simulink model "simSystem_v1"  (R2021b)
settings: Solver=VariableStepAuto  StartTime=0.0  StopTime=30  RelTol=1e-3
InitFcn:
  | initFcn
StopFcn:
  | stopFcn
values from neighbouring files (symbols this model uses):
  D_LIN = 1    [initFcn.m]
  D_QUAD = 1    [initFcn.m]
  M = M_RB + M_A    [initFcn.m]
  range = 2    [initFcn.m]
undefined symbols (not defined in the file or in its folder): B, I0, m, M_A, p, r_b_b, r_g_b, T
libraries: simulink x2, cstblocks x2, slpidlib x2, aerolibguid x1
settings Model: Creator=User  LastModifiedBy=saigon

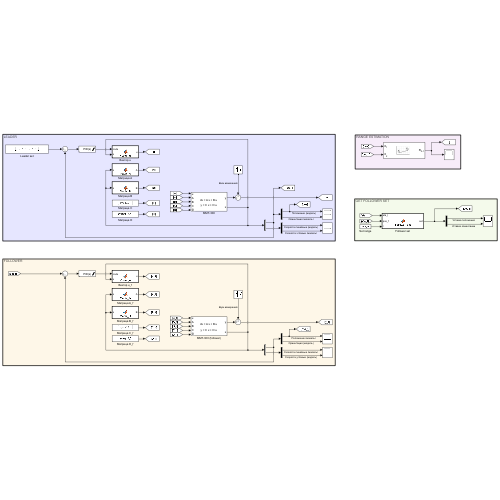
[thumbnail: Simulink's stored preview of the top-level diagram]
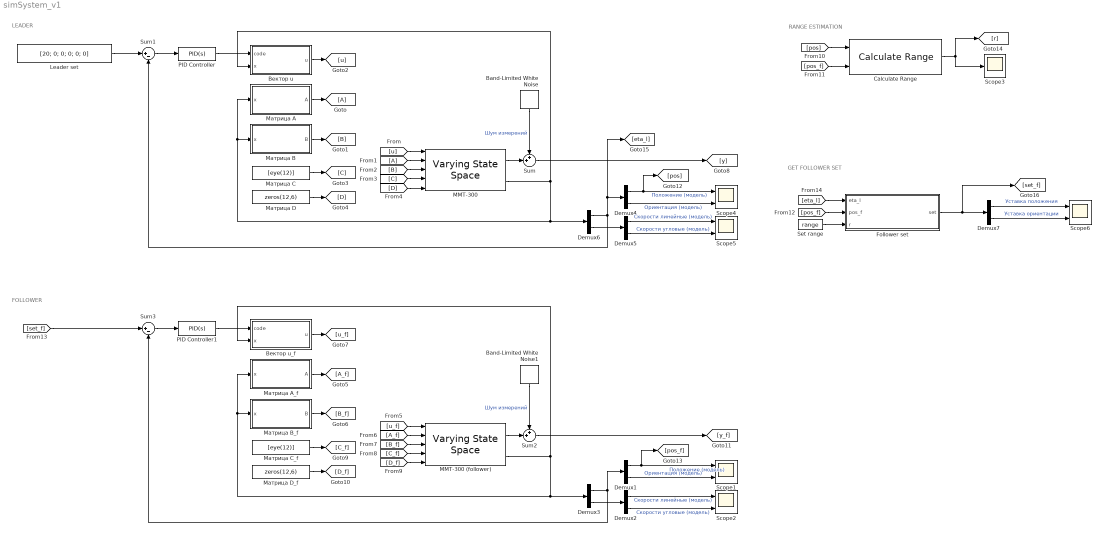
== system simSystem_v1 ==
  note: GET FOLLOWER SET
  note: RANGE ESTIMATION
  note: LEADER
  note: FOLLOWER
  Band-Limited White Noise : simulink/Sources/Band-Limited White Noise  Cov=[0.00000]  Ts=0.1  seed=[23341]
  Band-Limited White Noise1 : simulink/Sources/Band-Limited White Noise  Cov=[0.00000]  Ts=0.1  seed=[23341]
  Calculate Range : aerolibguid/Calculate Range
      settings: SourceProductBaseCode=AE
  Demux{1..7} (7 alike) : Demux  Outputs=2
  Follower set : MATLAB Function  TreatAsAtomicUnit=on
  Leader set : Constant  Value=[20; 0; 0; 0; 0; 0]
  MMT-300 : cstblocks/Linear Parameter Varying/Varying State Space  x0=zeros(12,1)  xNames=''  OutputX=on  OutputDX=off
  MMT-300 (follower) : cstblocks/Linear Parameter Varying/Varying State Space  x0=[-5;-5;0;0;0;0;zeros(6,1)]  xNames=''  OutputX=on  OutputDX=off
  PID Controller : slpidlib/PID Controller  Controller=PID  Form=Parallel  TimeDomain=Continuous-time  UseExternalTs=off  SampleTime=-1  IntegratorMethod=Forward Euler  FilterMethod=Forward Euler  ControllerParametersSource=internal  P=[100; 100; 100; 1500; 1500; 1500]  I=[0.5; 0.5; 0.5; 1; 1; 1]  D=[300; 300; 300; 400; 400; 400]  UseFilter=on  N=100  TunerSelectOption=Transfer Function Based (PID Tuner App)  InitialConditionSource=internal  InitialConditionForIntegrator=0  InitialConditionForFilter=0  DifferentiatorICPrevScaledInput=0  ExternalReset=none  TrackingMode=off  Kt=1  LimitOutput=on  SatLimitsSource=internal  UpperSaturationLimit=1000  LowerSaturationLimit=-1000  LinearizeAsGain=on  AntiWindupMode=none  Kb=1  POutMin=[]  POutMax=[]  IOutMin=[]  IOutMax=[]  DOutMin=[]  DOutMax=[]  NOutMin=[]  NOutMax=[]  SumOutMin=[]  SumOutMax=[]  SaturationOutMin=[]  SaturationOutMax=[]  PParamMin=[]  PParamMax=[]  IParamMin=[]  IParamMax=[]  DParamMin=[]  DParamMax=[]  NParamMin=[]  NParamMax=[]  KbParamMin=[]  KbParamMax=[]  KtParamMin=[]  KtParamMax=[]  KbOutMin=[]  KbOutMax=[]  KtOutMin=[]  KtOutMax=[]  IntegratorOutMin=[]  IntegratorOutMax=[]  FilterOutMin=[]  FilterOutMax=[]  SumI1OutMin=[]  SumI1OutMax=[]  SumI2OutMin=[]  SumI2OutMax=[]  SumI3OutMin=[]  SumI3OutMax=[]  SumI4OutMin=[]  SumI4OutMax=[]  SumDOutMin=[]  SumDOutMax=[]  DifferentiatorOutMin=[]  DifferentiatorOutMax=[]  FilterDiffOutCoefMin=[]  FilterDiffOutCoefMax=[]  ReciprocalOutMin=[]  ReciprocalOutMax=[]  SumDenOutMin=[]  SumDenOutMax=[]  SumNumOutMin=[]  SumNumOutMax=[]  DivideOutMin=[]  DivideOutMax=[]  UdiffTsProdOutMin=[]  UdiffTsProdOutMax=[]  NTsProdOutMin=[]  NTsProdOutMax=[]  UintegralTsProdOutMin=[]  UintegralTsProdOutMax=[]  UngainTsProdOutMin=[]  UngainTsProdOutMax=[]  IntegratorContinuousStateAttributes=''  IntegratorStateMustResolveToSignalObject=off  IntegratorRTWStateStorageClass=Auto  FilterContinuousStateAttributes=''  FilterStateMustResolveToSignalObject=off  FilterRTWStateStorageClass=Auto  ParallelPVariant=InternalParameters  IdealPVariant=Disabled  IVariant=InternalParameters  DVariant=InternalParameters  IntegratorVariant=Continuous  SatVariant=Enabled  AWVariant=Passthrough  PCopyVariant=Disabled  TRVariant=Disabled  FdbkBlocksVariant=Forward  IdealPFdbkVariant=Disabled  SatFdbkVariant=Disabled  DerivativeFilterVariant=ContFilter  NVariant=InternalParameters  NCopyVariant=Disabled  FilterICVariant=InternalICsFilter  IntegratorICVariant=InternalICs  ExternalResetVariant=Disabled  TRSumVariant=Passthrough  SumFdbkVariant=Disabled  SumVariant=Sum_PID  TsampFilterVariant=InternalTs  TsampNgainVariant=Passthrough  TsampIntegralVariant=Passthrough  ExternalSaturationOutDataTypeStr=Inherit: Same as second input
  PID Controller1 : slpidlib/PID Controller  Controller=PID  Form=Parallel  TimeDomain=Continuous-time  UseExternalTs=off  SampleTime=-1  IntegratorMethod=Forward Euler  FilterMethod=Forward Euler  ControllerParametersSource=internal  P=[100; 100; 100; 1500; 1500; 1500]  I=[0.5; 0.5; 0.5; 1; 1; 1]  D=[300; 300; 300; 400; 400; 400]  UseFilter=on  N=100  TunerSelectOption=Transfer Function Based (PID Tuner App)  InitialConditionSource=internal  InitialConditionForIntegrator=0  InitialConditionForFilter=0  DifferentiatorICPrevScaledInput=0  ExternalReset=none  TrackingMode=off  Kt=1  LimitOutput=on  SatLimitsSource=internal  UpperSaturationLimit=1000  LowerSaturationLimit=-1000  LinearizeAsGain=on  AntiWindupMode=none  Kb=1  POutMin=[]  POutMax=[]  IOutMin=[]  IOutMax=[]  DOutMin=[]  DOutMax=[]  NOutMin=[]  NOutMax=[]  SumOutMin=[]  SumOutMax=[]  SaturationOutMin=[]  SaturationOutMax=[]  PParamMin=[]  PParamMax=[]  IParamMin=[]  IParamMax=[]  DParamMin=[]  DParamMax=[]  NParamMin=[]  NParamMax=[]  KbParamMin=[]  KbParamMax=[]  KtParamMin=[]  KtParamMax=[]  KbOutMin=[]  KbOutMax=[]  KtOutMin=[]  KtOutMax=[]  IntegratorOutMin=[]  IntegratorOutMax=[]  FilterOutMin=[]  FilterOutMax=[]  SumI1OutMin=[]  SumI1OutMax=[]  SumI2OutMin=[]  SumI2OutMax=[]  SumI3OutMin=[]  SumI3OutMax=[]  SumI4OutMin=[]  SumI4OutMax=[]  SumDOutMin=[]  SumDOutMax=[]  DifferentiatorOutMin=[]  DifferentiatorOutMax=[]  FilterDiffOutCoefMin=[]  FilterDiffOutCoefMax=[]  ReciprocalOutMin=[]  ReciprocalOutMax=[]  SumDenOutMin=[]  SumDenOutMax=[]  SumNumOutMin=[]  SumNumOutMax=[]  DivideOutMin=[]  DivideOutMax=[]  UdiffTsProdOutMin=[]  UdiffTsProdOutMax=[]  NTsProdOutMin=[]  NTsProdOutMax=[]  UintegralTsProdOutMin=[]  UintegralTsProdOutMax=[]  UngainTsProdOutMin=[]  UngainTsProdOutMax=[]  IntegratorContinuousStateAttributes=''  IntegratorStateMustResolveToSignalObject=off  IntegratorRTWStateStorageClass=Auto  FilterContinuousStateAttributes=''  FilterStateMustResolveToSignalObject=off  FilterRTWStateStorageClass=Auto  ParallelPVariant=InternalParameters  IdealPVariant=Disabled  IVariant=InternalParameters  DVariant=InternalParameters  IntegratorVariant=Continuous  SatVariant=Enabled  AWVariant=Passthrough  PCopyVariant=Disabled  TRVariant=Disabled  FdbkBlocksVariant=Forward  IdealPFdbkVariant=Disabled  SatFdbkVariant=Disabled  DerivativeFilterVariant=ContFilter  NVariant=InternalParameters  NCopyVariant=Disabled  FilterICVariant=InternalICsFilter  IntegratorICVariant=InternalICs  ExternalResetVariant=Disabled  TRSumVariant=Passthrough  SumFdbkVariant=Disabled  SumVariant=Sum_PID  TsampFilterVariant=InternalTs  TsampNgainVariant=Passthrough  TsampIntegralVariant=Passthrough  ExternalSaturationOutDataTypeStr=Inherit: Same as second input
  Scope{1..2,4..6} (5 alike) : Scope  NumInputPorts=2
  Scope3 : Scope
  Set range : Constant  Value=range
  Sum : Sum  Inputs=++|
  Sum1 : Sum  Inputs=|+-
  Sum2 : Sum  Inputs=++|
  Sum3 : Sum  Inputs=|+-
  Вектор u : MATLAB Function  TreatAsAtomicUnit=on
  Вектор u_f : MATLAB Function  TreatAsAtomicUnit=on
  Матрица A : MATLAB Function  TreatAsAtomicUnit=on
  Матрица A_f : MATLAB Function  TreatAsAtomicUnit=on
  Матрица B : MATLAB Function  TreatAsAtomicUnit=on
  Матрица B_f : MATLAB Function  TreatAsAtomicUnit=on
  Матрица C : Constant  Value=[eye(12)]
  Матрица C_f : Constant  Value=[eye(12)]
  Матрица D : Constant  Value=zeros(12,6)
  Матрица D_f : Constant  Value=zeros(12,6)
  wires:
  MMT-300/1 -> Sum/2
  Band-Limited White Noise/1 -> Sum/1  "Шум измерений"
  Demux4/1 -> [pos], Scope4/1  "Положение (модель)"
  Demux4/2 -> Scope4/2  "Ориентация (модель)"
  Demux5/2 -> Scope5/2  "Скорости угловые (модель)"
  Demux5/1 -> Scope5/1  "Скорости линейные (модель)"
  Demux6/2 -> Demux5/1
  Матрица A/1(A) -> [A]
  Матрица B/1(B) -> [B]
  Вектор u/1(u) -> [u]
  Матрица C/1 -> [C]
  Матрица D/1 -> [D]
  [u] -> MMT-300/1
  [A] -> MMT-300/2
  [B] -> MMT-300/3
  [C] -> MMT-300/4
  [D] -> MMT-300/5
  MMT-300/2 -> Demux6/1, Матрица A/1(x), Матрица B/1(x), Вектор u/2(x)
  Sum/1 -> [y]
  Leader set/1 -> Sum1/1
  PID Controller/1 -> Вектор u/1(code)
  Sum1/1 -> PID Controller/1
  Sum3/1 -> PID Controller1/1
  PID Controller1/1 -> Вектор u_f/1(code)
  [set_f] -> Sum3/1
  Sum2/1 -> [y_f]
  MMT-300 (follower)/2 -> Вектор u_f/2(x), Матрица B_f/1(x), Матрица A_f/1(x), Demux3/1
  [D_f] -> MMT-300 (follower)/5
  [C_f] -> MMT-300 (follower)/4
  [B_f] -> MMT-300 (follower)/3
  [A_f] -> MMT-300 (follower)/2
  [u_f] -> MMT-300 (follower)/1
  Матрица D_f/1 -> [D_f]
  Матрица C_f/1 -> [C_f]
  Вектор u_f/1(u) -> [u_f]
  Матрица B_f/1(B) -> [B_f]
  Матрица A_f/1(A) -> [A_f]
  Demux3/1 -> Demux1/1, Sum3/2
  Demux3/2 -> Demux2/1
  Demux2/1 -> Scope2/1  "Скорости линейные (модель)"
  Demux2/2 -> Scope2/2  "Скорости угловые (модель)"
  Demux1/2 -> Scope1/2  "Ориентация (модель)"
  Demux1/1 -> [pos_f], Scope1/1  "Положение (модель)"
  Band-Limited White Noise1/1 -> Sum2/1  "Шум измерений"
  MMT-300 (follower)/1 -> Sum2/2
  [pos] -> Calculate Range/1
  [pos_f] -> Calculate Range/2
  Calculate Range/1 -> [r], Scope3/1
  [pos_f] -> Follower set/2(pos_f)
  Set range/1 -> Follower set/3(r)
  Demux6/1 -> Sum1/2, [eta_l], Demux4/1
  [eta_l] -> Follower set/1(eta_l)
  Follower set/1(set) -> [set_f], Demux7/1
  Demux7/2 -> Scope6/2  "Уставка ориентации"
  Demux7/1 -> Scope6/1  "Уставка положения"

== matlab function simSystem_v1/Вектор u_f ==
  data: code input [-127..127]; x input size=12; u output size=6; T parameter; p parameter; B parameter; m parameter; r_g_b parameter; r_b_b parameter
function u = Vector_u(code, x, T, p, B, m, r_g_b, r_b_b)
n = 6;
eta = x(1:n); 

%% РАСЧЕТ g(n)
x_g = r_g_b(1); y_g = r_g_b(2); z_g = r_g_b(3);
x_b = r_b_b(1); y_b = r_b_b(2); z_b = r_b_b(3);
g = @(eta)[ (m*9.81-B)*sin(eta(5)); 
           -(m*9.81-B)*cos(eta(5))*sin(eta(4)); 
           -(m*9.81-B)*cos(eta(5))*cos(eta(4));
           -(y_g*m*9.81-y_b*B)*cos(eta(5))*cos(eta(4)) + ...
              (z_g*m*9.81-z_b*B)*cos(eta(5))*sin(eta(4));
            (z_g*m*9.81-z_b*B)*sin(eta(5)) + ...
              (x_g*m*9.81-x_b*B)*cos(eta(5))*cos(eta(4));
           -(x_g*m*9.81-x_b*B)*cos(eta(5))*sin(eta(4)) - ...
              (y_g*m*9.81-y_b*B)*sin(eta(5)) ]; 


F = @(code)polyval(p,code);

f1 = @(code)[ F(code)*cos(deg2rad(22)); 
              0; 
              F(code)*sin(deg2rad(22)) ];
f2 = @(code)[ F(code)*cos(deg2rad(22)); 
              F(code)*sin(deg2rad(22));
              0 ];
f3 = @(code)[ F(code)*cos(deg2rad(22)); 
              0; 
              -F(code)*sin(deg2rad(22)) ];
f4 = @(code)[ F(code)*cos(deg2rad(22));  
              -F(code)*sin(deg2rad(22));
              0 ];
f5 = @(code)[ 0; 
              F(code); 
              0 ];
f6 = @(code)[ 0; 
              0; 
              -F(code) ];

r1 = T(1,:)'; 
r2 = T(2,:)'; 
r3 = T(3,:)';
r4 = T(4,:)';
r5 = T(5,:)';
r6 = T(6,:)';
tau1 = @(code)[ f1(code); cross(r1, f1(code)) ];
tau2 = @(code)[ f2(code); cross(r2, f2(code)) ];
tau3 = @(code)[ f3(code); cross(r3, f3(code)) ];
tau4 = @(code)[ f4(code); cross(r4, f4(code)) ];
tau5 = @(code)[ f5(code); cross(r5, f5(code)) ];
tau6 = @(code)[ f6(code); cross(r6, f6(code)) ];

tau_c = @(code)[ tau1(code(1)), tau2(code(2)), tau3(code(3)), ...
                 tau4(code(4)), tau5(code(5)), tau6(code(6)) ];

thruster_mask = [1, 1, 1, 1, 1, 1]';

%u = -g(eta) + tau_c(code) * thruster_mask;
u = -g(eta) + code;

== matlab function simSystem_v1/Матрица A_f ==
  data: x input size=12; A output size=[12 12]; M parameter; I0 parameter; r_g_b parameter; m parameter; r_b_b parameter; M_A parameter; D_LIN parameter; D_QUAD parameter
function A = Matrix_A(x, M, I0, r_g_b, m, r_b_b, M_A, D_LIN, D_QUAD)
n = 6;
eta = x(1:n); 
v = x(7:end);

%% ВСПОМОГАТЕЛЬНЫЕ ФУНКЦИИ
% преобразование в кососимметричную матрицу
S = @(x)([ 0 -x(3) x(2); x(3) 0 -x(1); -x(2) x(1) 0 ]); 

%% РАСЧЕТ ЯКОБИАНА
J_k_o = @(eta)[ 1  0           -sin(eta(5)); ...
                0  cos(eta(4))  cos(eta(5))*sin(eta(4)); ...
                0 -sin(eta(4))  cos(eta(5))*cos(eta(4)) ];
R_I_B = @(eta)[ cos(eta(6))*cos(eta(5))                                        sin(eta(6))*cos(eta(5))                                       -sin(eta(5)); ...
               -sin(eta(6))*cos(eta(4)) + cos(eta(6))*sin(eta(5))*sin(eta(4))  cos(eta(6))*cos(eta(4)) + sin(eta(6))*sin(eta(5))*sin(eta(4))  sin(eta(4))*cos(eta(5)); ...
                sin(eta(6))*sin(eta(4)) + cos(eta(6))*sin(eta(5))*cos(eta(4)) -cos(eta(6))*sin(eta(4)) + sin(eta(6))*sin(eta(5))*cos(eta(4))  cos(eta(4))*cos(eta(5)) ];
J = @(eta)[ R_I_B(eta) zeros(3); ...
            zeros(3)   J_k_o(eta) ];

%% РАСЧЕТ C(v)
% расчет C_RB(v)
%C_RB = @(v)([ zeros(3) -m*S(v(1:3)); -m*S(v(1:3)) -S(diag(I0).*v(4:end)) ]); 
C_RB = @(v)[ zeros(3)                           -m*S(v(1:3))-m*S(S(v(4:end))*r_g_b); ...
            -m*S(v(1:3))-m*S(S(v(4:end))*r_g_b)  m*S(S(v(1:3))*r_g_b)-S(I0*v(4:end)) ];
% расчет C_A(v)
diag_M_A = diag(M_A);
C_A = @(v)([ zeros(3) -S(diag_M_A(1:3).*v(1:3));
    -S(diag_M_A(1:3).*v(1:3)) -S(diag_M_A(4:end).*v(4:end))]);
% расчет C(v)
C = @(v)(C_RB(v) + C_A(v)); 
% M11 = M(1:3,1:3); M12 = M(1:3,4:6); M21 = M(4:6,1:3); M22 = M(4:6,4:6);
% C = @(v)[ zeros(3) -S(M11*v(1:3)+M12*v(4:6)); -S(M11*v(1:3)+M12*v(4:6)) -S(M21*v(1:3)+M22*v(4:6)) ];

%% РАСЧЕТ D(v)
%D = @(v)(abs(D_LIN) + abs(D_QUAD).*abs(v)); 
D = @(v)(zeros(6,6)); 

A = [zeros(n), J(eta)^-1;
     zeros(n), -M^-1 * ( C(v) + D(v) )];

== matlab function simSystem_v1/Матрица A ==
  data: x input size=12; A output size=[12 12]; M parameter; I0 parameter; r_g_b parameter; m parameter; r_b_b parameter; M_A parameter; D_LIN parameter; D_QUAD parameter
function A = Matrix_A(x, M, I0, r_g_b, m, r_b_b, M_A, D_LIN, D_QUAD)
n = 6;
eta = x(1:n); 
v = x(7:end);

%% ВСПОМОГАТЕЛЬНЫЕ ФУНКЦИИ
% преобразование в кососимметричную матрицу
S = @(x)([ 0 -x(3) x(2); x(3) 0 -x(1); -x(2) x(1) 0 ]); 

%% РАСЧЕТ ЯКОБИАНА
J_k_o = @(eta)[ 1  0           -sin(eta(5)); ...
                0  cos(eta(4))  cos(eta(5))*sin(eta(4)); ...
                0 -sin(eta(4))  cos(eta(5))*cos(eta(4)) ];
R_I_B = @(eta)[ cos(eta(6))*cos(eta(5))                                        sin(eta(6))*cos(eta(5))                                       -sin(eta(5)); ...
               -sin(eta(6))*cos(eta(4)) + cos(eta(6))*sin(eta(5))*sin(eta(4))  cos(eta(6))*cos(eta(4)) + sin(eta(6))*sin(eta(5))*sin(eta(4))  sin(eta(4))*cos(eta(5)); ...
                sin(eta(6))*sin(eta(4)) + cos(eta(6))*sin(eta(5))*cos(eta(4)) -cos(eta(6))*sin(eta(4)) + sin(eta(6))*sin(eta(5))*cos(eta(4))  cos(eta(4))*cos(eta(5)) ];
J = @(eta)[ R_I_B(eta) zeros(3); ...
            zeros(3)   J_k_o(eta) ];

%% РАСЧЕТ C(v)
% расчет C_RB(v)
%C_RB = @(v)([ zeros(3) -m*S(v(1:3)); -m*S(v(1:3)) -S(diag(I0).*v(4:end)) ]); 
C_RB = @(v)[ zeros(3)                           -m*S(v(1:3))-m*S(S(v(4:end))*r_g_b); ...
            -m*S(v(1:3))-m*S(S(v(4:end))*r_g_b)  m*S(S(v(1:3))*r_g_b)-S(I0*v(4:end)) ];
% расчет C_A(v)
diag_M_A = diag(M_A);
C_A = @(v)([ zeros(3) -S(diag_M_A(1:3).*v(1:3));
    -S(diag_M_A(1:3).*v(1:3)) -S(diag_M_A(4:end).*v(4:end))]);
% расчет C(v)
C = @(v)(C_RB(v) + C_A(v)); 
% M11 = M(1:3,1:3); M12 = M(1:3,4:6); M21 = M(4:6,1:3); M22 = M(4:6,4:6);
% C = @(v)[ zeros(3) -S(M11*v(1:3)+M12*v(4:6)); -S(M11*v(1:3)+M12*v(4:6)) -S(M21*v(1:3)+M22*v(4:6)) ];

%% РАСЧЕТ D(v)
%D = @(v)(abs(D_LIN) + abs(D_QUAD).*abs(v)); 
D = @(v)(zeros(6,6)); 

A = [zeros(n), J(eta)^-1;
     zeros(n), -M^-1 * ( C(v) + D(v) )];

== matlab function simSystem_v1/Матрица B ==
  data: x input size=12; B output size=[12 6]; M parameter
function B = Matrix_B(x, M)
n = 6;
B = [zeros(n); M^-1];

== matlab function simSystem_v1/Вектор u ==
  data: code input [-127..127]; x input size=12; u output size=6; T parameter; p parameter; B parameter; m parameter; r_g_b parameter; r_b_b parameter
function u = Vector_u(code, x, T, p, B, m, r_g_b, r_b_b)
n = 6;
eta = x(1:n); 

%% РАСЧЕТ g(n)
x_g = r_g_b(1); y_g = r_g_b(2); z_g = r_g_b(3);
x_b = r_b_b(1); y_b = r_b_b(2); z_b = r_b_b(3);
g = @(eta)[ (m*9.81-B)*sin(eta(5)); 
           -(m*9.81-B)*cos(eta(5))*sin(eta(4)); 
           -(m*9.81-B)*cos(eta(5))*cos(eta(4));
           -(y_g*m*9.81-y_b*B)*cos(eta(5))*cos(eta(4)) + ...
              (z_g*m*9.81-z_b*B)*cos(eta(5))*sin(eta(4));
            (z_g*m*9.81-z_b*B)*sin(eta(5)) + ...
              (x_g*m*9.81-x_b*B)*cos(eta(5))*cos(eta(4));
           -(x_g*m*9.81-x_b*B)*cos(eta(5))*sin(eta(4)) - ...
              (y_g*m*9.81-y_b*B)*sin(eta(5)) ]; 


F = @(code)polyval(p,code);

f1 = @(code)[ F(code)*cos(deg2rad(22)); 
              0; 
              F(code)*sin(deg2rad(22)) ];
f2 = @(code)[ F(code)*cos(deg2rad(22)); 
              F(code)*sin(deg2rad(22));
              0 ];
f3 = @(code)[ F(code)*cos(deg2rad(22)); 
              0; 
              -F(code)*sin(deg2rad(22)) ];
f4 = @(code)[ F(code)*cos(deg2rad(22));  
              -F(code)*sin(deg2rad(22));
              0 ];
f5 = @(code)[ 0; 
              F(code); 
              0 ];
f6 = @(code)[ 0; 
              0; 
              -F(code) ];

r1 = T(1,:)'; 
r2 = T(2,:)'; 
r3 = T(3,:)';
r4 = T(4,:)';
r5 = T(5,:)';
r6 = T(6,:)';
tau1 = @(code)[ f1(code); cross(r1, f1(code)) ];
tau2 = @(code)[ f2(code); cross(r2, f2(code)) ];
tau3 = @(code)[ f3(code); cross(r3, f3(code)) ];
tau4 = @(code)[ f4(code); cross(r4, f4(code)) ];
tau5 = @(code)[ f5(code); cross(r5, f5(code)) ];
tau6 = @(code)[ f6(code); cross(r6, f6(code)) ];

tau_c = @(code)[ tau1(code(1)), tau2(code(2)), tau3(code(3)), ...
                 tau4(code(4)), tau5(code(5)), tau6(code(6)) ];

thruster_mask = [1, 1, 1, 1, 1, 1]';

%u = -g(eta) + tau_c(code) * thruster_mask;
u = -g(eta) + code;

== matlab function simSystem_v1/Матрица B_f ==
  data: x input size=12; B output size=[12 6]; M parameter
function B = Matrix_B(x, M)
n = 6;
B = [zeros(n); M^-1];

== matlab function simSystem_v1/Follower set ==
  data: eta_l input size=6 [-127..127]; pos_f input size=3; set output size=6; r input
function set = Follower_set(eta_l, pos_f, r)
pos_l = eta_l(1:3);
set = zeros(6,1);
set(3) = pos_l(3);
set(6) = eta_l(6);

P1 = @(pos_l, pos_f, r) [ pos_l(1) + (r*(pos_f(1)-pos_l(1))) / sqrt((pos_f(1)-pos_l(1))^2 + (pos_f(2)-pos_l(2))^2); ...
                          pos_l(2) + (r*(pos_f(2)-pos_l(2))) / sqrt((pos_f(1)-pos_l(1))^2 + (pos_f(2)-pos_l(2))^2) ];
P2 = @(pos_l, pos_f, r) [ pos_l(1) - (r*(pos_f(1)-pos_l(1))) / sqrt((pos_f(1)-pos_l(1))^2 + (pos_f(2)-pos_l(2))^2); ...
                          pos_l(2) - (r*(pos_f(2)-pos_l(2))) / sqrt((pos_f(1)-pos_l(1))^2 + (pos_f(2)-pos_l(2))^2) ];
% Две возможные точки
p1 = P1(pos_l, pos_f, r);
p2 = P2(pos_l, pos_f, r);
% Две нормы
n = [ norm(p1 - pos_f(1:2)); ... 
      norm(p2 - pos_f(1:2)) ];
% Ищем минимальную
[~, idx] = min(n);
if (idx == 1)
    set(1) = p1(1); set(2) = p1(2);
else
    set(1) = p2(1); set(2) = p2(1);
end
